simulink model "fuzzySystems"  (R2017a)
settings: Solver=VariableStepAuto  StartTime=0.0  StopTime=5  RelTol=1e-3
values from neighbouring files (symbols this model uses):
  K = 50    [lab.m]
  Tau = 0.1    [lab.m]
libraries: fuzblock x1
settings Model: Creator=abd el rahman  LastModifiedBy=abd el rahman

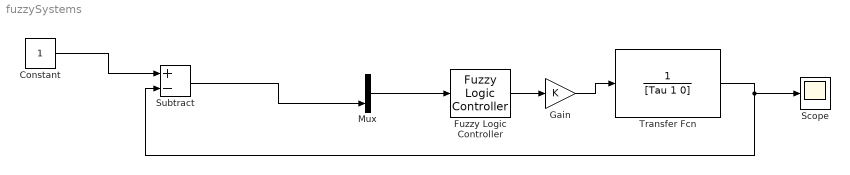
== system fuzzySystems ==
  Constant : Constant
  Fuzzy Logic Controller : fuzblock/Fuzzy Logic  Controller  fis='MyController.fis'
  Gain : Gain  Gain=K
  Mux : Mux  Inputs=2
  Scope : Scope
  Subtract : Sum  Inputs=+-
  Transfer Fcn : TransferFcn  Denominator=[Tau 1 0]
  wires:
  Mux/1 -> Fuzzy Logic Controller/1
  Transfer Fcn/1 -> Subtract/2, Scope/1
  Constant/1 -> Subtract/1
  Subtract/1 -> Mux/2
  Fuzzy Logic Controller/1 -> Gain/1
  Gain/1 -> Transfer Fcn/1
